simulink model "NavigationRocketPlant"  (R2025b)
settings: Solver=ode5  StartTime=0.0  StopTime=350  RelTol=1e-3
PostLoadFcn:
  | addpath('settings/')
  | addpath('settings/environment/')
  | 
  | run sensorSettings.m
InitFcn:
  | run(fullfile(fileparts(get_param(bdroot,'FileName')),'..','rocketPlantMain.m'))
values from neighbouring files (symbols this model uses):
  ba0 = zeros(3,1)    [rocketPlantMain.m]
  bg0 = zeros(3,1)    [rocketPlantMain.m]
  LLA0 = [Rocket.Latitude; Rocket.Longitude; Rocket.AltitudeMSL]    [rocketPlantMain.m]
  p0 = zeros(3,1)    [rocketPlantMain.m]
  P0 = zeros(15,15)    [rocketPlantMain.m]
  q0 = RocketInitialState(7:10)    [rocketPlantMain.m]
  RocketInitialState = rocketPlantInitialize(Rocket)    [rocketPlantMain.m]
  stationaryTime = Rocket.IgnitionTime    [rocketPlantMain.m]
  v0 = zeros(3,1)    [rocketPlantMain.m]
undefined symbols (not defined in the file or in its folder): DiscIntNeverNeededParam, dspblkCoreblockFVToolHelper, Environment, gcbh, GNSSConfig, GNSSInitialState, MEKF, pressure0, Rocket, Sensor, Weather
libraries: simulink x2, dspmathops x1
(part 1 of 3)
settings Model: Creator=wujia  LastModifiedBy=wujia

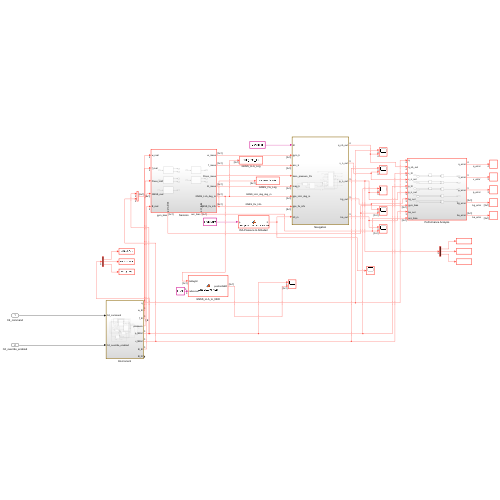
[thumbnail: Simulink's stored preview of the top-level diagram]
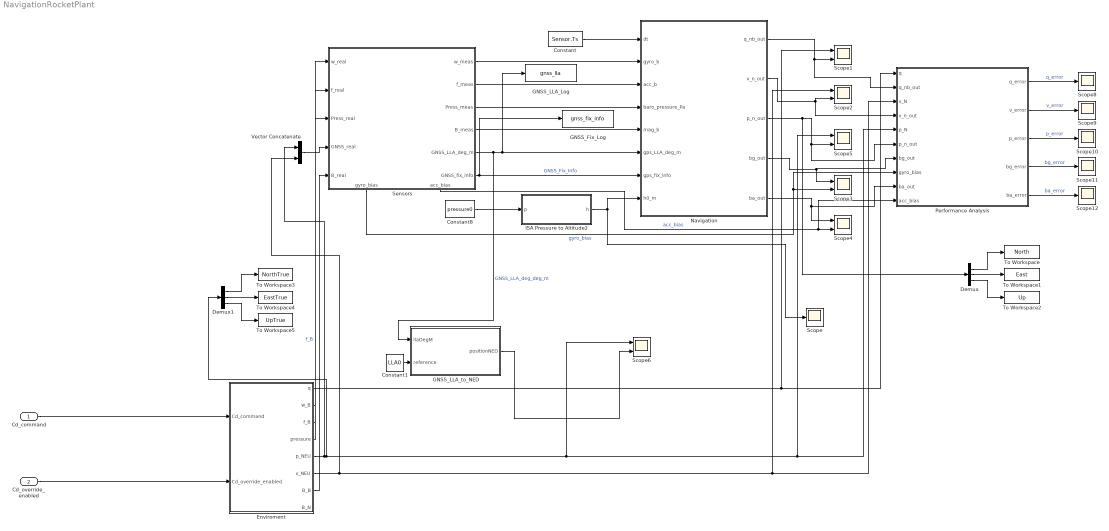
== system NavigationRocketPlant ==
  Cd_command : Inport  OutDataTypeStr=double  PortDimensions=1  SampleTime=Rocket.Ts  Interpolate=off
  Cd_override_enabled : Inport  Port=2  OutDataTypeStr=double  PortDimensions=1  SampleTime=Rocket.Ts  Interpolate=off
  Constant : Constant  Value=Sensor.Ts
  Constant1 : Constant  Value=LLA0
  Constant8 : Constant  Value=pressure0
  Demux : Demux  Outputs=3
  Demux1 : Demux  Outputs=3
  Enviroment : Subsystem
  GNSS_Fix_Log : ToWorkspace  VariableName=gnss_fix_info  SaveFormat=Timeseries  SampleTime=-1
  GNSS_LLA_Log : ToWorkspace  VariableName=gnss_lla  SaveFormat=Timeseries  SampleTime=-1
  GNSS_LLA_to_NED : MATLAB Function  TreatAsAtomicUnit=on
  ISA Pressure to Altitude2 : MATLAB Function  TreatAsAtomicUnit=on
  Navigation : Subsystem
  Performance Analysis : Subsystem
  Scope{,8..12} (6 alike) : Scope
      Scope settings: ActiveDisplayYMinimum=-1  ActiveDisplayYMaximum=1  DataLoggingVariableName=ScopeData18
      Scope10 settings: ActiveDisplayYMinimum=-43.238898122556691  ActiveDisplayYMaximum=55.159382964966909  DataLoggingVariableName=ScopeData12
      Scope11 settings: ActiveDisplayYMinimum=-0.047372671781054559  ActiveDisplayYMaximum=0.023017615287449465  DataLoggingVariableName=ScopeData13
      Scope12 settings: ActiveDisplayYMinimum=-0.56247304441899837  ActiveDisplayYMaximum=1.1440559822181913  DataLoggingVariableName=ScopeData14
      Scope8 settings: ActiveDisplayYMinimum=-2.4024992579145321  ActiveDisplayYMaximum=2.4014240203083954  DataLoggingVariableName=ScopeData6
      Scope9 settings: ActiveDisplayYMinimum=-73.4449521246089  ActiveDisplayYMaximum=67.234314688531754  DataLoggingVariableName=ScopeData8
  Scope{1..6} (6 alike) : Scope  NumInputPorts=2
      Scope1 settings: ActiveDisplayYMinimum=-1.2880369168448469  ActiveDisplayYMaximum=1.3322786485025644
      Scope2 settings: ActiveDisplayYMinimum=-66.391402806495847  ActiveDisplayYMaximum=368.05030772718362  DataLoggingVariableName=ScopeData2
      Scope3 settings: ActiveDisplayYMinimum=-0.019866552939701122  ActiveDisplayYMaximum=0.055696216205846576  DataLoggingVariableName=ScopeData3
      Scope4 settings: ActiveDisplayYMinimum=-0.56108731493308794  ActiveDisplayYMaximum=1.1446707904167028  DataLoggingVariableName=ScopeData4
      Scope5 settings: ActiveDisplayYMinimum=-703.59600028849377  ActiveDisplayYMaximum=4675.4737500320552  DataLoggingVariableName=ScopeData5
      Scope6 settings: ActiveDisplayYMinimum=-4.2977064407464418  ActiveDisplayYMaximum=41.562392937860714  DataLoggingVariableName=ScopeData7
  Sensors : Subsystem
      settings: PortSchema="{\"entries\":[{\"content\":{\"sides\":[{\"content\":{\"connectorIds\":[\"In1\",\"In2\",\"In3\",\"In4\",\"In5\"]},\"type\":\"ConnectorPlacement.EquallySpacedRectSide\",\"uuid\":\"7549c628-8b7d-407c-a68e-245c0e15f536\"},{\"content\":{\"connectorIds\":[\"Out1\",\"Out2\",\"Out3\",\"Out4\",\"Out5\",\"Out6\"],\"side\":\"RIGHT\"},\"type\":\"ConnectorPlacement.EquallySpacedRectSide\",\"uuid\":\"d27d0e7f-3d86-4e84-80b8-20c86293b7bf\"},{\"content\":{\"side\":\"TOP\"},\"type\":\"ConnectorPlacement.EquallySpacedRectSide\",\"uuid\":\"44c73c2c-96b0-4d3a-9d50-da6ca6099998\"},{\"content\":{\"connectorIds\":[\"Out7\",\"Out8\"],\"side\":\"BOTTOM\"},\"type\":\"ConnectorPlacement.EquallySpacedRectSide\",\"uuid\":\"8107c7d0-06da-4640-bff8-8544b9179788\"}]},\"type\":\"ConnectorPlacement.EquallySpacedConnector\",\"uuid\":\"f9c24899-cf40-457b-80ff-0dc7874e17ca\"}],\"packageUris\":[\"http://schema.mathworks.com/mf0/Connector/R2020b\"],\"version\":\"1.0\"}"
  To Workspace : ToWorkspace  VariableName=North  SaveFormat=Structure  SampleTime=-1
      settings: Save2DSignal=2-D array (concatenate along first dimension)
  To Workspace1 : ToWorkspace  VariableName=East  SaveFormat=Structure  SampleTime=-1
      settings: Save2DSignal=2-D array (concatenate along first dimension)
  To Workspace2 : ToWorkspace  VariableName=Up  SaveFormat=Structure  SampleTime=-1
      settings: Save2DSignal=2-D array (concatenate along first dimension)
  To Workspace3 : ToWorkspace  VariableName=NorthTrue  SaveFormat=Structure  SampleTime=-1
      settings: Save2DSignal=2-D array (concatenate along first dimension)
  To Workspace4 : ToWorkspace  VariableName=EastTrue  SaveFormat=Structure  SampleTime=-1
      settings: Save2DSignal=2-D array (concatenate along first dimension)
  To Workspace5 : ToWorkspace  VariableName=UpTrue  SaveFormat=Structure  SampleTime=-1
      settings: Save2DSignal=2-D array (concatenate along first dimension)
  Vector Concatenate : Concatenate  Mode=Multidimensional array
  wires:
  Sensors/4(B_meas) -> Navigation/5(mag_b)
  Sensors/3(Press_meas) -> Navigation/4(baro_pressure_Pa)
  Constant8/1 -> ISA Pressure to Altitude2/1(p)
  Sensors/7(gyro_bias) -> Performance Analysis/8(gyro_bias), Scope3/2  "gyro_bias"
  Sensors/8(acc_bias) -> Performance Analysis/10(acc_bias), Scope4/2  "acc_bias"
  Sensors/1(w_meas) -> Navigation/2(gyro_b)
  Constant/1 -> Navigation/1(dt)
  ISA Pressure to Altitude2/1(h) -> Scope/1, Navigation/8(h0_m)
  Navigation/1(q_nb_out) -> Performance Analysis/2(q_nb_out), Scope1/2
  Navigation/4(bg_out) -> Performance Analysis/7(bg_out), Scope3/1
  Navigation/5(ba_out) -> Scope4/1, Performance Analysis/9(ba_out)
  Vector Concatenate/1 -> Sensors/4(GNSS_real)
  Performance Analysis/1(q_error) -> Scope8/1  "q_error"
  Performance Analysis/2(v_error) -> Scope9/1  "v_error"
  Performance Analysis/5(ba_error) -> Scope12/1  "ba_error"
  Performance Analysis/4(bg_error) -> Scope11/1  "bg_error"
  Performance Analysis/3(p_error) -> Scope10/1  "p_error"
  Sensors/2(f_meas) -> Navigation/3(acc_b)
  Demux/1 -> To Workspace/1
  Demux/3 -> To Workspace2/1
  Demux/2 -> To Workspace1/1
  Demux1/1 -> To Workspace3/1
  Demux1/2 -> To Workspace4/1
  Demux1/3 -> To Workspace5/1
  Navigation/2(v_n_out) -> Performance Analysis/4(v_n_out), Scope2/2
  Navigation/3(p_n_out) -> Demux/1, Performance Analysis/6(p_n_out), Scope5/2
  Sensors/6(GNSS_fix_info) -> GNSS_Fix_Log/1, Navigation/7(gps_fix_info)  "GNSS_Fix_Info"
  Constant1/1 -> GNSS_LLA_to_NED/2(reference)
  GNSS_LLA_to_NED/1(positionNED) -> Scope6/2
  Sensors/5(GNSS_LLA_deg_m) -> Navigation/6(gps_LLA_deg_m), GNSS_LLA_Log/1, GNSS_LLA_to_NED/1(llaDegM)  "GNSS_LLA_deg_deg_m"
  Enviroment/2(w_B) -> Sensors/1(w_real)
  Enviroment/3(f_B) -> Sensors/2(f_real)  "f_B"
  Enviroment/7(B_B) -> Sensors/5(B_real)
  Enviroment/4(pressure) -> Sensors/3(Press_real)
  Enviroment/6(v_NEU) -> Performance Analysis/3(v_N), Scope2/1, Vector Concatenate/2
  Enviroment/1(q) -> Performance Analysis/1(q), Scope1/1
  Enviroment/5(p_NEU) -> Performance Analysis/5(p_N), Scope5/1, Scope6/1, Demux1/1, Vector Concatenate/1
  Cd_command/1 -> Enviroment/1(Cd_command)
  Cd_override_enabled/1 -> Enviroment/2(Cd_override_enabled)

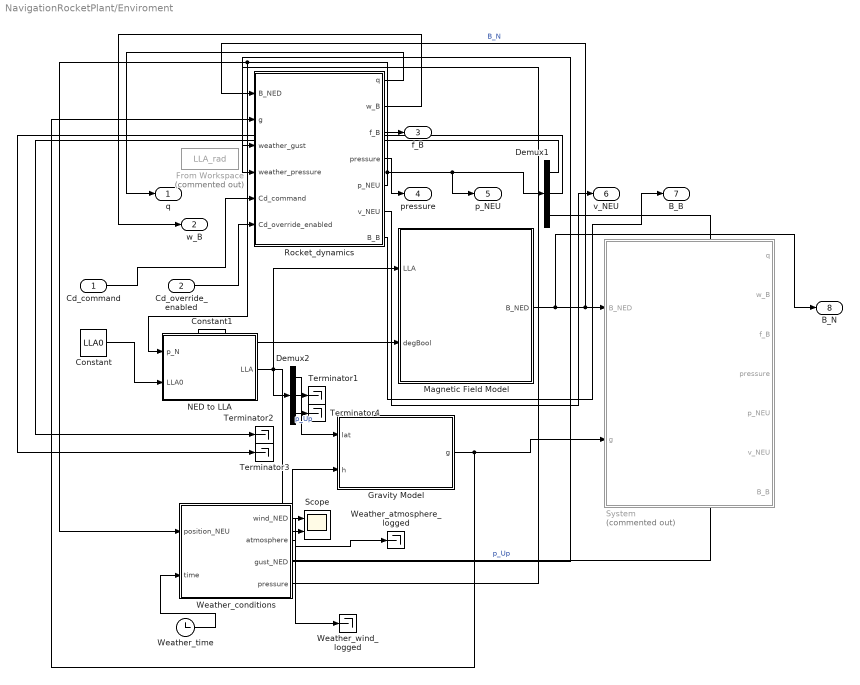
== system NavigationRocketPlant/Enviroment ==
  Cd_command : Inport  PortDimensions=1  SampleTime=Rocket.Ts
  Cd_override_enabled : Inport  Port=2  PortDimensions=1  SampleTime=Rocket.Ts
  Constant : Constant  Value=LLA0  VectorParams1D=off
  Constant1 : Constant  Value=0
  Demux1 : Demux  Outputs=3
  Demux2 : Demux  Outputs=3
  From Workspace : FromWorkspace  Commented=on  VariableName=LLA_rad
  Gravity Model : Subsystem
  Magnetic Field Model : Subsystem
  NED to LLA : MATLAB Function  TreatAsAtomicUnit=on
  Rocket_dynamics : Subsystem
  Scope : Scope  NumInputPorts=2
      settings: ActiveDisplayYMinimum=-1  ActiveDisplayYMaximum=1  DataLoggingVariableName=ScopeData9
  System : Subsystem  Description=Preserved CSV reference; inactive in physics-driven model. Original CSV model remains in the recovery artifact.  Commented=on
  Terminator{1..4} (4 alike) : Terminator
  Weather_atmosphere_logged : Terminator
  Weather_conditions : Subsystem
  Weather_time : Clock
  Weather_wind_logged : Terminator
  q : Outport
  w_B : Outport  Port=2
  f_B : Outport  Port=3
  pressure : Outport  Port=4
  p_NEU : Outport  Port=5
  v_NEU : Outport  Port=6
  B_B : Outport  Port=7
  B_N : Outport  Port=8
  wires:
  Demux2/2 -> Terminator1/1
  Demux2/3 -> Terminator4/1  "p_Up"
  Demux2/1 -> Gravity Model/1(lat)
  Demux1/3 -> Gravity Model/2(h)  "p_Up"
  Demux1/1 -> Terminator2/1
  Demux1/2 -> Terminator3/1
  Weather_conditions/2(atmosphere) -> Weather_atmosphere_logged/1
  Cd_override_enabled/1 -> Rocket_dynamics/6(Cd_override_enabled)
  Cd_command/1 -> Rocket_dynamics/5(Cd_command)
  Rocket_dynamics/7(B_B) -> B_B/1
  Rocket_dynamics/6(v_NEU) -> v_NEU/1
  Rocket_dynamics/5(p_NEU) -> Demux1/1, p_NEU/1, NED to LLA/1(p_N), Weather_conditions/1(position_NEU)
  Rocket_dynamics/4(pressure) -> pressure/1
  Rocket_dynamics/3(f_B) -> f_B/1
  Rocket_dynamics/2(w_B) -> w_B/1
  Rocket_dynamics/1(q) -> q/1
  Gravity Model/1(g) -> Rocket_dynamics/2(g), System/2(g)
  Magnetic Field Model/1(B_NED) -> Rocket_dynamics/1(B_NED), System/1(B_NED), B_N/1  "B_N"
  Weather_time/1 -> Weather_conditions/2(time)
  Weather_conditions/3(gust_NED) -> Rocket_dynamics/3(weather_gust)
  Weather_conditions/4(pressure) -> Rocket_dynamics/4(weather_pressure)
  Weather_conditions/1(wind_NED) -> Weather_wind_logged/1
  NED to LLA/1(LLA) -> Scope/2, Scope/1, Magnetic Field Model/1(LLA), Demux2/1
  Constant/1 -> NED to LLA/2(LLA0)
  Constant1/1 -> Magnetic Field Model/2(degBool)

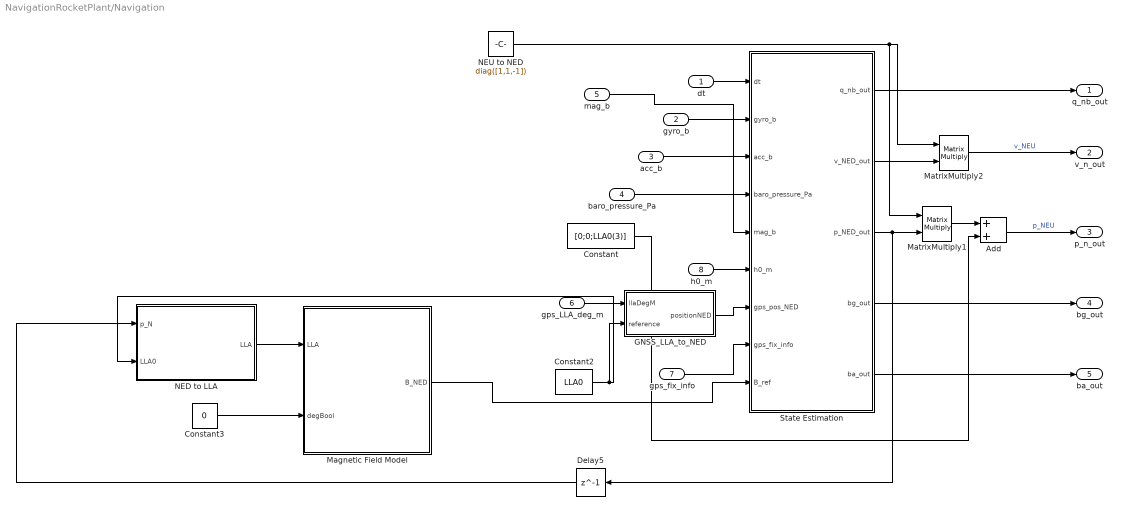
== system NavigationRocketPlant/Navigation ==
  dt : Inport
  gyro_b : Inport  Port=2
  acc_b : Inport  Port=3
  baro_pressure_Pa : Inport  Port=4
  mag_b : Inport  Port=5
  gps_LLA_deg_m : Inport  Port=6
  gps_fix_info : Inport  Port=7
  h0_m : Inport  Port=8
  Add : Sum
  Constant : Constant  Value=[0;0;LLA0(3)]
  Constant2 : Constant  Value=LLA0
  Constant3 : Constant  Value=0
  Delay5 : Delay  DelayLength=1  InitialCondition=p0
  GNSS_LLA_to_NED : MATLAB Function  TreatAsAtomicUnit=on
  Magnetic Field Model : Subsystem
  MatrixMultiply1 : Product  Multiplication=Matrix(*)
  MatrixMultiply2 : Product  Multiplication=Matrix(*)
  NED to LLA : MATLAB Function  TreatAsAtomicUnit=on
  NEU to NED : Constant  Value=diag([1,1,-1])
  State Estimation : Subsystem
  q_nb_out : Outport
  v_n_out : Outport  Port=2
  p_n_out : Outport  Port=3
  bg_out : Outport  Port=4
  ba_out : Outport  Port=5
  wires:
  MatrixMultiply2/1 -> v_n_out/1  "v_NEU"
  MatrixMultiply1/1 -> Add/1
  Constant3/1 -> Magnetic Field Model/2(degBool)
  NED to LLA/1(LLA) -> Magnetic Field Model/1(LLA)
  Delay5/1 -> NED to LLA/1(p_N)
  Add/1 -> p_n_out/1  "p_NEU"
  Constant/1 -> Add/2
  NEU to NED/1 -> MatrixMultiply2/1, MatrixMultiply1/1
  gps_fix_info/1 -> State Estimation/8(gps_fix_info)
  GNSS_LLA_to_NED/1(positionNED) -> State Estimation/7(gps_pos_NED)
  gps_LLA_deg_m/1 -> GNSS_LLA_to_NED/1(llaDegM)
  mag_b/1 -> State Estimation/5(mag_b)
  Constant2/1 -> GNSS_LLA_to_NED/2(reference), NED to LLA/2(LLA0)
  State Estimation/5(ba_out) -> ba_out/1
  State Estimation/4(bg_out) -> bg_out/1
  State Estimation/3(p_NED_out) -> MatrixMultiply1/2, Delay5/1
  State Estimation/2(v_NED_out) -> MatrixMultiply2/2
  State Estimation/1(q_nb_out) -> q_nb_out/1
  dt/1 -> State Estimation/1(dt)
  acc_b/1 -> State Estimation/3(acc_b)
  gyro_b/1 -> State Estimation/2(gyro_b)
  h0_m/1 -> State Estimation/6(h0_m)
  baro_pressure_Pa/1 -> State Estimation/4(baro_pressure_Pa)
  Magnetic Field Model/1(B_NED) -> State Estimation/9(B_ref)

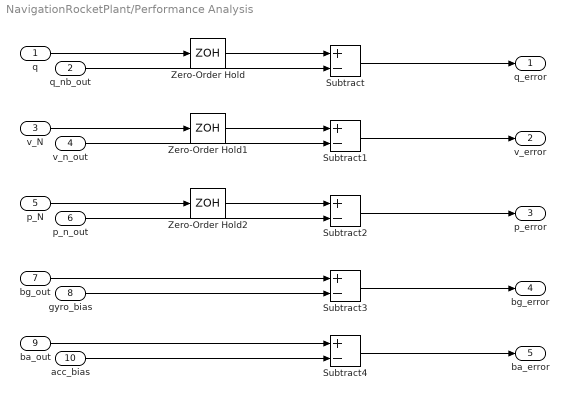
== system NavigationRocketPlant/Performance Analysis ==
  q : Inport
  q_nb_out : Inport  Port=2
  v_N : Inport  Port=3
  v_n_out : Inport  Port=4
  p_N : Inport  Port=5
  p_n_out : Inport  Port=6
  bg_out : Inport  Port=7
  gyro_bias : Inport  Port=8
  ba_out : Inport  Port=9
  acc_bias : Inport  Port=10
  Subtract{,1..4} (5 alike) : Sum  Inputs=+-
  Zero-Order Hold : ZeroOrderHold  SampleTime=Sensor.Ts
  Zero-Order Hold1 : ZeroOrderHold  SampleTime=-1
  Zero-Order Hold2 : ZeroOrderHold  SampleTime=-1
  q_error : Outport
  v_error : Outport  Port=2
  p_error : Outport  Port=3
  bg_error : Outport  Port=4
  ba_error : Outport  Port=5
  wires:
  q/1 -> Zero-Order Hold/1
  q_nb_out/1 -> Subtract/2
  v_n_out/1 -> Subtract1/2
  v_N/1 -> Zero-Order Hold1/1
  p_n_out/1 -> Subtract2/2
  p_N/1 -> Zero-Order Hold2/1
  bg_out/1 -> Subtract3/1
  gyro_bias/1 -> Subtract3/2
  ba_out/1 -> Subtract4/1
  acc_bias/1 -> Subtract4/2
  Zero-Order Hold1/1 -> Subtract1/1
  Zero-Order Hold2/1 -> Subtract2/1
  Subtract/1 -> q_error/1
  Subtract1/1 -> v_error/1
  Subtract2/1 -> p_error/1
  Subtract3/1 -> bg_error/1
  Subtract4/1 -> ba_error/1
  Zero-Order Hold/1 -> Subtract/1

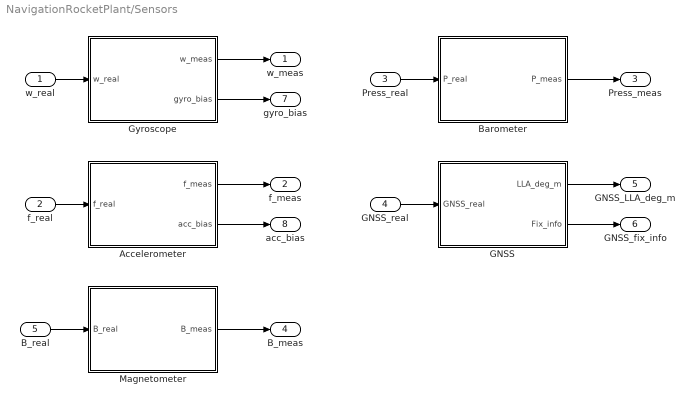
== system NavigationRocketPlant/Sensors ==
  w_real : Inport
  f_real : Inport  Port=2
  Press_real : Inport  Port=3
  GNSS_real : Inport  Port=4
  B_real : Inport  Port=5
  Accelerometer : Subsystem
  Barometer : Subsystem
  GNSS : Subsystem
  Gyroscope : Subsystem
  Magnetometer : Subsystem
  w_meas : Outport
  f_meas : Outport  Port=2
  Press_meas : Outport  Port=3
  B_meas : Outport  Port=4
  GNSS_LLA_deg_m : Outport  Description=Latitude [deg], longitude [deg], ellipsoid height [m].  Port=5
  GNSS_fix_info : Outport  Description=Fresh/valid/time/age/metric covariance/status; no velocity output.  Port=6
  gyro_bias : Outport  Port=7
  acc_bias : Outport  Port=8
  wires:
  B_real/1 -> Magnetometer/1(B_real)
  Magnetometer/1(B_meas) -> B_meas/1
  w_real/1 -> Gyroscope/1(w_real)
  f_real/1 -> Accelerometer/1(f_real)
  Accelerometer/1(f_meas) -> f_meas/1
  Gyroscope/1(w_meas) -> w_meas/1
  Barometer/1(P_meas) -> Press_meas/1
  Press_real/1 -> Barometer/1(P_real)
  GNSS_real/1 -> GNSS/1(GNSS_real)
  GNSS/1(LLA_deg_m) -> GNSS_LLA_deg_m/1
  GNSS/2(Fix_info) -> GNSS_fix_info/1
  Accelerometer/2(acc_bias) -> acc_bias/1
  Gyroscope/2(gyro_bias) -> gyro_bias/1

== system NavigationRocketPlant/Enviroment/Gravity Model ==
  lat : Inport
  h : Inport  Port=2
  MATLAB Function : MATLAB Function  TreatAsAtomicUnit=on
  MATLAB Function1 : MATLAB Function  TreatAsAtomicUnit=on
  Scope : Scope  NumInputPorts=2
      settings: ActiveDisplayYMinimum=9.7899742881861069  ActiveDisplayYMaximum=9.8055275433313476  DataLoggingVariableName=ScopeData19
  g : Outport
  wires:
  MATLAB Function/1(g) -> Scope/1
  h/1 -> MATLAB Function1/1(h), MATLAB Function/1(h)
  lat/1 -> MATLAB Function1/2(lat)
  MATLAB Function1/1(g_n) -> Scope/2, g/1

== system NavigationRocketPlant/Enviroment/Magnetic Field Model ==
  LLA : Inport
  degBool : Inport  Port=2
  Constant : Constant  Value=13
  MATLAB Function1 : MATLAB Function  Commented=on  TreatAsAtomicUnit=on
  Magnetic Field Model : MATLAB Function  TreatAsAtomicUnit=on
  Terminator : Terminator
  Terminator1 : Terminator
  g : Constant  Value=Environment.IGRF13.g
  h : Constant  Value=Environment.IGRF13.h
  order : Constant  Value=Environment.IGRF13.order
  B_NED : Outport
  wires:
  Magnetic Field Model/1(B_ECEF) -> Terminator1/1
  Magnetic Field Model/2(B_NED) -> B_NED/1
  g/1 -> Magnetic Field Model/2(g)
  order/1 -> ?
  h/1 -> Magnetic Field Model/3(h)
  LLA/1 -> Magnetic Field Model/1(LLA)
  Magnetic Field Model/3(B_sph) -> Terminator/1
  degBool/1 -> Magnetic Field Model/7(degBool)
  Constant/1 -> Magnetic Field Model/4(Nmax)

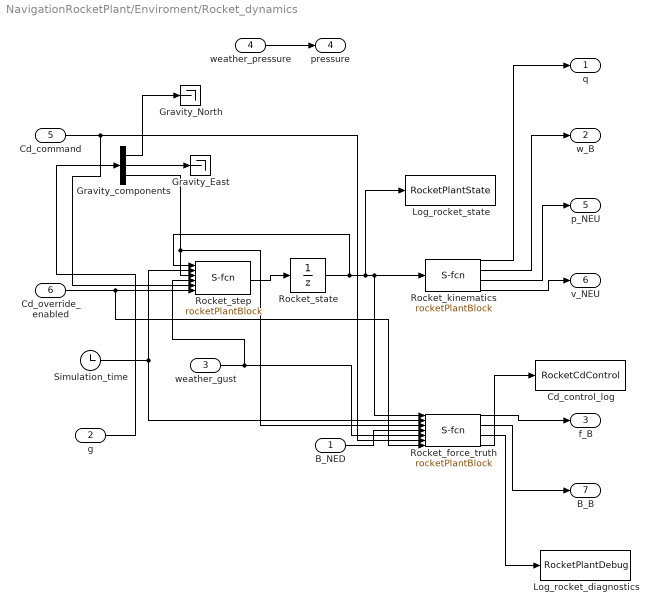
== system NavigationRocketPlant/Enviroment/Rocket_dynamics ==
  B_NED : Inport
  g : Inport  Port=2
  weather_gust : Inport  Port=3
  weather_pressure : Inport  Port=4
  Cd_command : Inport  Port=5  PortDimensions=1  SampleTime=Rocket.Ts
  Cd_override_enabled : Inport  Port=6  PortDimensions=1  SampleTime=Rocket.Ts
  Cd_control_log : ToWorkspace  VariableName=RocketCdControl  SaveFormat=Timeseries  SampleTime=-1
  Gravity_East : Terminator
  Gravity_North : Terminator
  Gravity_components : Demux  Outputs=3
  Log_rocket_diagnostics : ToWorkspace  VariableName=RocketPlantDebug  SaveFormat=Timeseries  SampleTime=-1
  Log_rocket_state : ToWorkspace  VariableName=RocketPlantState  SaveFormat=Timeseries  SampleTime=-1
  Rocket_force_truth : M-S-Function  FunctionName=rocketPlantBlock  Parameters=Rocket,3,Weather
  Rocket_kinematics : M-S-Function  FunctionName=rocketPlantBlock  Parameters=Rocket,2,Weather
  Rocket_state : UnitDelay  InitialCondition=RocketInitialState  SampleTime=Rocket.Ts  HasFrameUpgradeWarning=on
  Rocket_step : M-S-Function  FunctionName=rocketPlantBlock  Parameters=Rocket,1,Weather
  Simulation_time : Clock
  q : Outport
  w_B : Outport  Port=2
  f_B : Outport  Port=3
  pressure : Outport  Port=4
  p_NEU : Outport  Port=5
  v_NEU : Outport  Port=6
  B_B : Outport  Port=7
  wires:
  Rocket_force_truth/3 -> Log_rocket_diagnostics/1
  Rocket_force_truth/2 -> B_B/1
  Rocket_force_truth/1 -> f_B/1
  Rocket_kinematics/4 -> v_NEU/1
  Rocket_kinematics/3 -> p_NEU/1
  Rocket_kinematics/2 -> w_B/1
  Rocket_kinematics/1 -> q/1
  B_NED/1 -> Rocket_force_truth/4
  Rocket_step/1 -> Rocket_state/1
  g/1 -> Gravity_components/1
  Simulation_time/1 -> Rocket_step/2, Rocket_force_truth/2
  Rocket_state/1 -> Rocket_kinematics/1, Rocket_force_truth/1, Log_rocket_state/1, Rocket_step/1
  Gravity_components/3 -> Rocket_force_truth/3, Rocket_step/3
  Gravity_components/2 -> Gravity_East/1
  Gravity_components/1 -> Gravity_North/1
  weather_pressure/1 -> pressure/1
  weather_gust/1 -> Rocket_step/4, Rocket_force_truth/5
  Rocket_force_truth/4 -> Cd_control_log/1
  Cd_override_enabled/1 -> Rocket_force_truth/7, Rocket_step/6
  Cd_command/1 -> Rocket_force_truth/6, Rocket_step/5

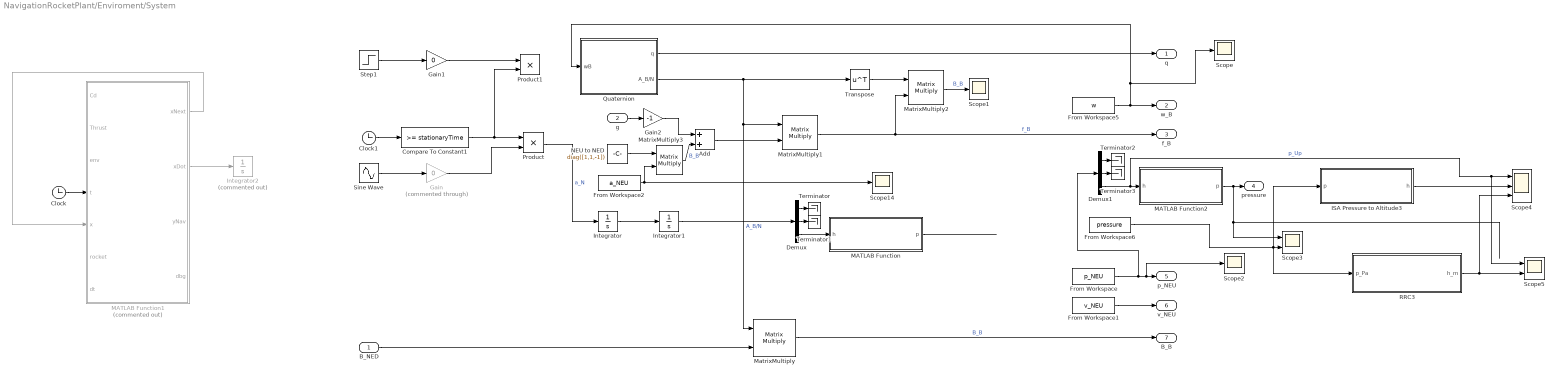
== system NavigationRocketPlant/Enviroment/System ==
  B_NED : Inport
  g : Inport  Port=2
  Add : Sum
  Clock : Clock
  Clock1 : Clock
  Compare To Constant1 : simulink/Logic and Bit Operations/Compare To Constant  relop=>=  const=stationaryTime  OutDataTypeStr=uint8
  Demux : Demux  Outputs=3
  Demux1 : Demux  Outputs=3
  From Workspace : FromWorkspace  VariableName=p_NEU  SampleTime=0.02
  From Workspace1 : FromWorkspace  VariableName=v_NEU  SampleTime=0.02
  From Workspace2 : FromWorkspace  VariableName=a_NEU  SampleTime=0.02
  From Workspace5 : FromWorkspace  VariableName=w  SampleTime=0.02
  From Workspace6 : FromWorkspace  VariableName=pressure  SampleTime=0.02
  Gain : Gain  Commented=through  Gain=0
  Gain1 : Gain  Gain=0
  Gain2 : Gain  Gain=-1
  ISA Pressure to Altitude3 : MATLAB Function  TreatAsAtomicUnit=on
  Integrator : Integrator  InitialCondition=v0
  Integrator1 : Integrator  InitialCondition=p0
  Integrator2 : Integrator  Commented=on
  MATLAB Function : MATLAB Function  TreatAsAtomicUnit=on
  MATLAB Function1 : MATLAB Function  Commented=on  TreatAsAtomicUnit=on
  MATLAB Function2 : MATLAB Function  TreatAsAtomicUnit=on
  MatrixMultiply{,1..3} (4 alike) : Product  Multiplication=Matrix(*)
  NEU to NED : Constant  Value=diag([1,1,-1])
  Product : Product
  Product1 : Product
  "Quaternion " : Subsystem
  RRC3 : MATLAB Function  TreatAsAtomicUnit=on
  Scope{,1..2,14} (4 alike) : Scope
      Scope settings: ActiveDisplayYMinimum=-1.6045475791322781E-7  ActiveDisplayYMaximum=2.6814536853544749E-7
      Scope1 settings: ActiveDisplayYMinimum=-185.19167567929276  ActiveDisplayYMaximum=161.84122591706938  DataLoggingVariableName=ScopeData15
      Scope14 settings: ActiveDisplayYMinimum=-34.139290674344366  ActiveDisplayYMaximum=25.55163695065562  DataLoggingVariableName=ScopeData20
      Scope2 settings: ActiveDisplayYMinimum=-1  ActiveDisplayYMaximum=1  DataLoggingVariableName=ScopeData16
  Scope3 : Scope  NumInputPorts=2
      settings: ActiveDisplayYMinimum=56252.912155082136  ActiveDisplayYMaximum=99152.104181642775  DataLoggingVariableName=ScopeData17
  Scope4 : Scope  NumInputPorts=3
      settings: ActiveDisplayYMinimum=3919.4855259572764  ActiveDisplayYMaximum=3932.9364289417367  DataLoggingVariableName=ScopeData17
  Scope5 : Scope  NumInputPorts=2
      settings: ActiveDisplayYMinimum=496.42915312500008  ActiveDisplayYMaximum=4542.137621875  DataLoggingVariableName=ScopeData11
  Sine Wave : Sin  Amplitude=[1;1;1]  Frequency=[0.1;0.2;0.3]  SampleTime=0  VectorParams1D=off
  Step1 : Step  Time=stationaryTime  After=[0.1;0.5;0.3]  SampleTime=0  VectorParams1D=off
  Terminator{,1..3} (4 alike) : Terminator
  Transpose : Math  Operator=transpose
  q : Outport
  w_B : Outport  Port=2
  f_B : Outport  Port=3
  pressure : Outport  Port=4
  p_NEU : Outport  Port=5
  v_NEU : Outport  Port=6
  B_B : Outport  Port=7
  wires:
  Integrator1/1 -> Demux/1
  B_NED/1 -> MatrixMultiply/2
  Clock1/1 -> Compare To Constant1/1
  Product/1 -> Integrator/1  "a_N"
  g/1 -> Gain2/1
  Step1/1 -> Gain1/1
  MatrixMultiply/1 -> B_B/1  "B_B"
  Integrator/1 -> Integrator1/1
  "Quaternion "/2("A_B/N ") -> Transpose/1, MatrixMultiply/1, MatrixMultiply1/1  "A_B/N"
  Compare To Constant1/1 -> Product1/2, Product/1
  Add/1 -> MatrixMultiply1/2
  Demux/1 -> Terminator/1
  Sine Wave/1 -> Gain/1
  Demux/3 -> MATLAB Function/1(h)
  MatrixMultiply1/1 -> MatrixMultiply2/2, f_B/1  "f_B"
  Gain/1 -> Product/2
  Demux/2 -> Terminator1/1
  MATLAB Function1/2(xDot) -> Integrator2/1
  From Workspace6/1 -> RRC3/1(p_Pa), ISA Pressure to Altitude3/1(p), Scope3/2
  From Workspace1/1 -> v_NEU/1
  From Workspace2/1 -> Scope14/1, MatrixMultiply3/2
  "Quaternion "/1(q) -> q/1
  Transpose/1 -> MatrixMultiply2/1
  MatrixMultiply2/1 -> Scope1/1  "B_B"
  Demux1/2 -> Terminator3/1
  Demux1/1 -> Terminator2/1
  MATLAB Function2/1(p) -> Scope3/1, pressure/1
  Gain1/1 -> Product1/1
  From Workspace/1 -> Demux1/1, p_NEU/1, Scope2/1
  From Workspace5/1 -> Scope/1, "Quaternion "/1(wB), w_B/1
  NEU to NED/1 -> MatrixMultiply3/1
  MatrixMultiply3/1 -> Add/2  "B_B"
  ISA Pressure to Altitude3/1(h) -> Scope4/2
  Demux1/3 -> Scope5/1, Scope4/1, MATLAB Function2/1(h)  "p_Up"
  RRC3/1(h_m) -> Scope4/3, Scope5/2
  Gain2/1 -> Add/1
  MATLAB Function1/1(xNext) -> MATLAB Function1/5(x)
  Clock/1 -> MATLAB Function1/4(t)
  MATLAB Function/1(p) -> ?

== system NavigationRocketPlant/Enviroment/Weather_conditions ==
  position_NEU : Inport
  time : Inport  Port=2
  Atmosphere_components : Demux  Outputs=5
  Density_log_only : Terminator
  Humidity_log_only : Terminator
  Log_weather_truth : ToWorkspace  VariableName=WeatherTruth  SaveFormat=Timeseries  SampleTime=-1
  Sound_speed_log_only : Terminator
  Temperature_log_only : Terminator
  Weather_log_vector : Mux  Inputs=3
  Weather_truth : M-S-Function  FunctionName=rocketWeatherBlock  Parameters=Rocket,Weather,Rocket.Ts
  wind_NED : Outport
  atmosphere : Outport  Port=2
  gust_NED : Outport  Port=3
  pressure : Outport  Port=4
  wires:
  Weather_truth/3 -> gust_NED/1, Weather_log_vector/3
  Weather_truth/2 -> Atmosphere_components/1, Weather_log_vector/2, atmosphere/1
  Weather_truth/1 -> Weather_log_vector/1, wind_NED/1
  time/1 -> Weather_truth/2
  position_NEU/1 -> Weather_truth/1
  Weather_log_vector/1 -> Log_weather_truth/1
  Atmosphere_components/1 -> Density_log_only/1
  Atmosphere_components/2 -> pressure/1
  Atmosphere_components/3 -> Sound_speed_log_only/1
  Atmosphere_components/4 -> Temperature_log_only/1
  Atmosphere_components/5 -> Humidity_log_only/1

== system NavigationRocketPlant/Navigation/Magnetic Field Model ==
  LLA : Inport
  degBool : Inport  Port=2
  Magnetic Field Model : MATLAB Function  TreatAsAtomicUnit=on
  Terminator : Terminator
  Terminator1 : Terminator
  g : Constant  Value=Environment.IGRF13.g
  h : Constant  Value=Environment.IGRF13.h
  order : Constant  Value=Environment.IGRF13.order
  B_NED : Outport
  wires:
  Magnetic Field Model/1(B_ECEF) -> Terminator1/1
  Magnetic Field Model/2(B_NED) -> B_NED/1
  g/1 -> Magnetic Field Model/2(g)
  order/1 -> Magnetic Field Model/4(Nmax)
  h/1 -> Magnetic Field Model/3(h)
  LLA/1 -> Magnetic Field Model/1(LLA)
  Magnetic Field Model/3(B_sph) -> Terminator/1
  degBool/1 -> Magnetic Field Model/5(degBool)

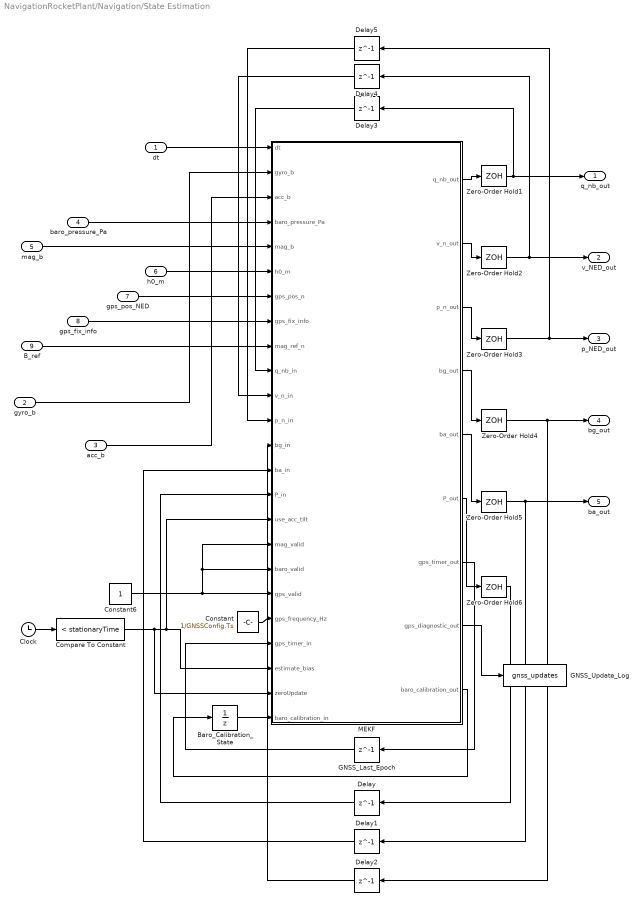
== system NavigationRocketPlant/Navigation/State Estimation ==
  dt : Inport
  gyro_b : Inport  Port=2
  acc_b : Inport  Port=3
  baro_pressure_Pa : Inport  Port=4
  mag_b : Inport  Port=5
  h0_m : Inport  Port=6
  gps_pos_NED : Inport  Port=7
  gps_fix_info : Inport  Port=8
  B_ref : Inport  Port=9
  Baro_Calibration_State : UnitDelay  InitialCondition=[0;0]  SampleTime=Sensor.Ts  HasFrameUpgradeWarning=on
  Clock : Clock
  Compare To Constant : simulink/Logic and Bit Operations/Compare To Constant  relop=<  const=stationaryTime  OutDataTypeStr=boolean
  Constant : Constant  Value=1/GNSSConfig.Ts
  Constant6 : Constant
  Delay : Delay  DelayLength=1  InitialCondition=P0  SampleTime=Sensor.Ts
  Delay1 : Delay  DelayLength=1  InitialCondition=ba0  SampleTime=Sensor.Ts
  Delay2 : Delay  DelayLength=1  InitialCondition=bg0  SampleTime=Sensor.Ts
  Delay3 : Delay  DelayLength=1  InitialCondition=q0  SampleTime=Sensor.Ts
  Delay4 : Delay  DelayLength=1  InitialCondition=v0  SampleTime=Sensor.Ts
  Delay5 : Delay  DelayLength=1  InitialCondition=p0  SampleTime=Sensor.Ts
  GNSS_Last_Epoch : Delay  DelayLength=1  InitialCondition=-1  InputProcessing=Columns as channels (frame based)
  GNSS_Update_Log : ToWorkspace  VariableName=gnss_updates  SaveFormat=Timeseries  SampleTime=-1
  MEKF : MATLAB Function  TreatAsAtomicUnit=on
  Zero-Order Hold{1..6} (6 alike) : ZeroOrderHold  SampleTime=-1
  q_nb_out : Outport
  v_NED_out : Outport  Port=2
  p_NED_out : Outport  Port=3
  bg_out : Outport  Port=4
  ba_out : Outport  Port=5
  wires:
  Clock/1 -> Compare To Constant/1
  Zero-Order Hold1/1 -> Delay3/1, q_nb_out/1
  Zero-Order Hold2/1 -> v_NED_out/1, Delay4/1
  Zero-Order Hold3/1 -> p_NED_out/1, Delay5/1
  Zero-Order Hold4/1 -> Delay2/1, bg_out/1
  Zero-Order Hold5/1 -> Delay1/1, ba_out/1
  Zero-Order Hold6/1 -> Delay/1
  Baro_Calibration_State/1 -> MEKF/24(baro_calibration_in)
  MEKF/9(baro_calibration_out) -> Baro_Calibration_State/1
  MEKF/8(gps_diagnostic_out) -> GNSS_Update_Log/1
  gyro_b/1 -> MEKF/2(gyro_b)
  acc_b/1 -> MEKF/3(acc_b)
  MEKF/6(P_out) -> Zero-Order Hold6/1
  Constant/1 -> MEKF/20(gps_frequency_Hz)
  GNSS_Last_Epoch/1 -> MEKF/21(gps_timer_in)
  MEKF/7(gps_timer_out) -> GNSS_Last_Epoch/1
  Delay1/1 -> MEKF/14(ba_in)
  Constant6/1 -> MEKF/17(mag_valid), MEKF/18(baro_valid), MEKF/19(gps_valid)
  Delay/1 -> MEKF/15(P_in)
  mag_b/1 -> MEKF/5(mag_b)
  Delay5/1 -> MEKF/12(p_n_in)
  MEKF/3(p_n_out) -> Zero-Order Hold3/1
  gps_pos_NED/1 -> MEKF/7(gps_pos_n)
  h0_m/1 -> MEKF/6(h0_m)
  baro_pressure_Pa/1 -> MEKF/4(baro_pressure_Pa)
  gps_fix_info/1 -> MEKF/8(gps_fix_info)
  B_ref/1 -> MEKF/9(mag_ref_n)
  MEKF/1(q_nb_out) -> Zero-Order Hold1/1
  dt/1 -> MEKF/1(dt)
  Compare To Constant/1 -> MEKF/16(use_acc_tilt), MEKF/22(estimate_bias), MEKF/23(zeroUpdate)
  Delay2/1 -> MEKF/13(bg_in)
  MEKF/4(bg_out) -> Zero-Order Hold4/1
  Delay4/1 -> MEKF/11(v_n_in)
  MEKF/5(ba_out) -> Zero-Order Hold5/1
  MEKF/2(v_n_out) -> Zero-Order Hold2/1
  Delay3/1 -> MEKF/10(q_nb_in)

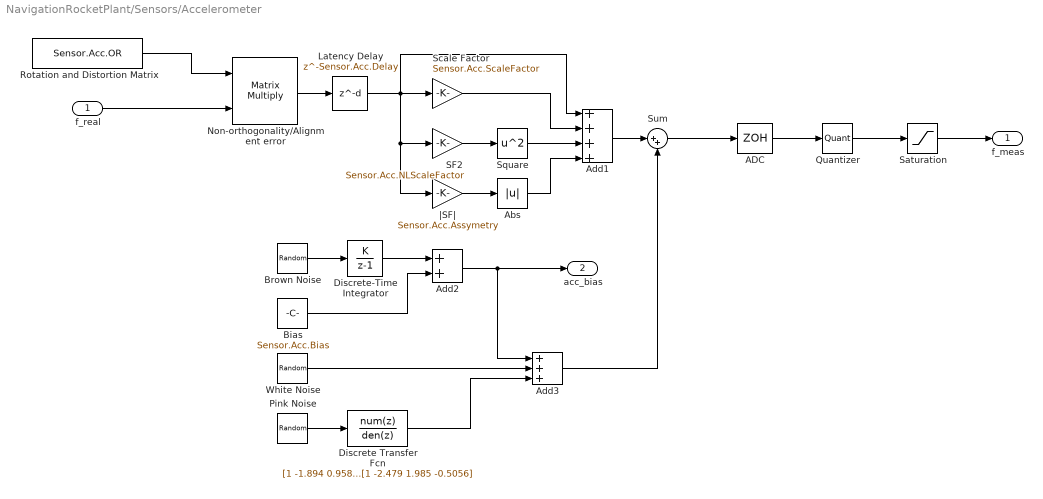
== system NavigationRocketPlant/Sensors/Accelerometer ==
  f_real : Inport
  ADC : ZeroOrderHold  SampleTime=Sensor.Acc.Ts
  Abs : Abs  SaturateOnIntegerOverflow=off
  Add1 : Sum  Inputs=++++
  Add2 : Sum
  Add3 : Sum  Inputs=+++
  Bias : Constant  Value=Sensor.Acc.Bias  VectorParams1D=off  SampleTime=Sensor.Acc.Ts
  Brown Noise : RandomNumber  Mean=Sensor.Acc.Noise.Brown.Mean  Variance=Sensor.Acc.Noise.Brown.Variance  Seed=Sensor.Acc.Noise.Brown.Seed  SampleTime=Sensor.Acc.Ts  VectorParams1D=off
  Discrete Transfer Fcn : DiscreteTransferFcn  LoadFcn=dspblkCoreblockFVToolHelper(gcbh,'load');  Numerator=[1 -1.894 0.9586 -0.06213]  Denominator=[1 -2.479 1.985 -0.5056]
      settings: CopyFcn=dspblkCoreblockFVToolHelper(gcbh,'copy');  DeleteFcn=dspblkCoreblockFVToolHelper(gcbh,'close');  ModelCloseFcn=dspblkCoreblockFVToolHelper(gcbh,'close');  PreSaveFcn=dspblkCoreblockFVToolHelper(gcbh,'presave');  PostSaveFcn=dspblkCoreblockFVToolHelper(gcbh,'postsave');  CloseFcn=dspblkCoreblockFVToolHelper(gcbh,'close');
  Discrete-Time Integrator : DiscreteIntegrator  IntegratorMethod=Accumulation: Forward Euler  SampleTime=Sensor.Acc.Ts  ICPrevOutput=DiscIntNeverNeededParam  ICPrevScaledInput=DiscIntNeverNeededParam
  Latency Delay : Delay  DelayLength=Sensor.Acc.Delay  SampleTime=Sensor.Acc.Ts
  Non-orthogonality/Alignment error : Product  Multiplication=Matrix(*)
  Pink Noise : RandomNumber  Mean=Sensor.Acc.Noise.Pink.Mean  Variance=Sensor.Acc.Noise.Pink.Variance  Seed=Sensor.Acc.Noise.Pink.Seed  SampleTime=Sensor.Acc.Ts  VectorParams1D=off
  Quantizer : Quantizer  QuantizationInterval=Sensor.Acc.Quant
  Rotation and Distortion Matrix : Constant  Value=Sensor.Acc.OR
  SF2 : Gain  Gain=Sensor.Acc.NLScaleFactor
  "Saturation " : Saturate  UpperLimit=Sensor.Acc.UpperLim  LowerLimit=Sensor.Acc.LowerLim
  Scale Factor : Gain  Gain=Sensor.Acc.ScaleFactor
  Square : Math  Operator=square
  Sum : Sum  Inputs=|++
  White Noise : RandomNumber  Mean=Sensor.Acc.Noise.White.Mean  Variance=Sensor.Acc.Noise.White.Variance  Seed=Sensor.Acc.Noise.White.Seed  SampleTime=Sensor.Acc.Ts  VectorParams1D=off
  |SF| : Gain  Gain=Sensor.Acc.Assymetry
  f_meas : Outport
  acc_bias : Outport  Port=2
  wires:
  f_real/1 -> Non-orthogonality/Alignment error/2
  Sum/1 -> ADC/1
  White Noise/1 -> Add3/2
  Bias/1 -> Add2/2
  Add3/1 -> Sum/2
  Brown Noise/1 -> Discrete-Time Integrator/1
  Discrete-Time Integrator/1 -> Add2/1
  ADC/1 -> Quantizer/1
  Latency Delay/1 -> Add1/1, SF2/1, |SF|/1, Scale Factor/1
  "Saturation "/1 -> f_meas/1
  Pink Noise/1 -> Discrete Transfer Fcn/1
  Discrete Transfer Fcn/1 -> Add3/3
  SF2/1 -> Square/1
  |SF|/1 -> Abs/1
  Scale Factor/1 -> Add1/2
  Square/1 -> Add1/3
  Abs/1 -> Add1/4
  Add1/1 -> Sum/1
  Quantizer/1 -> "Saturation "/1
  Non-orthogonality/Alignment error/1 -> Latency Delay/1
  Rotation and Distortion Matrix/1 -> Non-orthogonality/Alignment error/1
  Add2/1 -> acc_bias/1, Add3/1

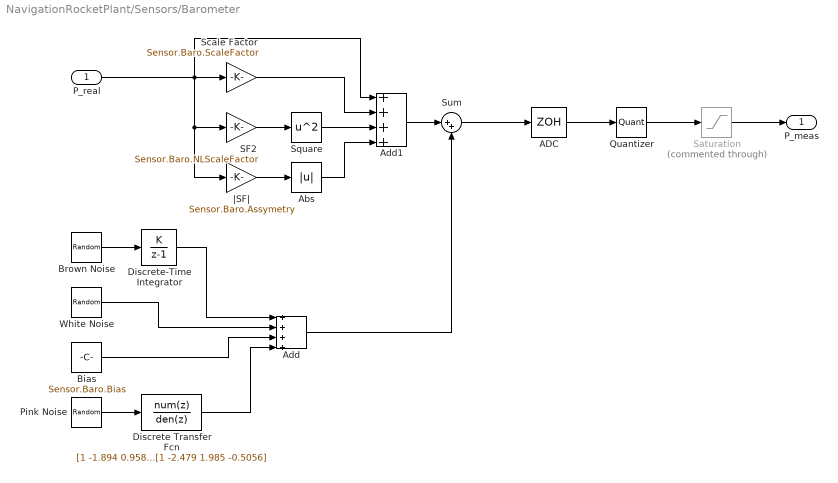
== system NavigationRocketPlant/Sensors/Barometer ==
  P_real : Inport
  ADC : ZeroOrderHold  SampleTime=Sensor.Baro.Ts
  Abs : Abs  SaturateOnIntegerOverflow=off
  Add : Sum  Inputs=++++
  Add1 : Sum  Inputs=++++
  Bias : Constant  Value=Sensor.Baro.Bias
  Brown Noise : RandomNumber  Mean=Sensor.Baro.Noise.Brown.Mean  Variance=Sensor.Baro.Noise.Brown.Variance  Seed=Sensor.Baro.Noise.Brown.Seed  SampleTime=Sensor.Baro.Ts
  Discrete Transfer Fcn : DiscreteTransferFcn  LoadFcn=dspblkCoreblockFVToolHelper(gcbh,'load');  Numerator=[1 -1.894 0.9586 -0.06213]  Denominator=[1 -2.479 1.985 -0.5056]
      settings: CopyFcn=dspblkCoreblockFVToolHelper(gcbh,'copy');  DeleteFcn=dspblkCoreblockFVToolHelper(gcbh,'close');  ModelCloseFcn=dspblkCoreblockFVToolHelper(gcbh,'close');  PreSaveFcn=dspblkCoreblockFVToolHelper(gcbh,'presave');  PostSaveFcn=dspblkCoreblockFVToolHelper(gcbh,'postsave');  CloseFcn=dspblkCoreblockFVToolHelper(gcbh,'close');
  Discrete-Time Integrator : DiscreteIntegrator  IntegratorMethod=Accumulation: Forward Euler  SampleTime=Sensor.Baro.Ts  ICPrevOutput=DiscIntNeverNeededParam  ICPrevScaledInput=DiscIntNeverNeededParam
  Pink Noise : RandomNumber  Mean=Sensor.Baro.Noise.Pink.Mean  Variance=Sensor.Baro.Noise.Pink.Variance  Seed=Sensor.Baro.Noise.Pink.Seed  SampleTime=Sensor.Baro.Ts
  Quantizer : Quantizer  QuantizationInterval=Sensor.Baro.Quant
  SF2 : Gain  Gain=Sensor.Baro.NLScaleFactor
  "Saturation " : Saturate  Commented=through  UpperLimit=Sensor.Baro.UpperLim  LowerLimit=Sensor.Baro.LowerLim
  Scale Factor : Gain  Gain=Sensor.Baro.ScaleFactor
  Square : Math  Operator=square
  Sum : Sum  Inputs=|++
  White Noise : RandomNumber  Mean=Sensor.Baro.Noise.White.Mean  Variance=Sensor.Baro.Noise.White.Variance  Seed=Sensor.Baro.Noise.White.Seed  SampleTime=Sensor.Baro.Ts
  |SF| : Gain  Gain=Sensor.Baro.Assymetry
  P_meas : Outport
  wires:
  Sum/1 -> ADC/1
  White Noise/1 -> Add/2
  Bias/1 -> Add/3
  Add/1 -> Sum/2
  Brown Noise/1 -> Discrete-Time Integrator/1
  Discrete-Time Integrator/1 -> Add/1
  ADC/1 -> Quantizer/1
  P_real/1 -> Add1/1, SF2/1, |SF|/1, Scale Factor/1
  "Saturation "/1 -> P_meas/1
  Pink Noise/1 -> Discrete Transfer Fcn/1
  Discrete Transfer Fcn/1 -> Add/4
  SF2/1 -> Square/1
  |SF|/1 -> Abs/1
  Scale Factor/1 -> Add1/2
  Square/1 -> Add1/3
  Abs/1 -> Add1/4
  Add1/1 -> Sum/1
  Quantizer/1 -> "Saturation "/1

== system NavigationRocketPlant/Sensors/GNSS ==
  GNSS_real : Inport
  GNSS_Clock : DigitalClock  SampleTime=GNSSConfig.Ts/GNSSConfig.TransportSubsteps
  GNSS_Consume : MATLAB Function  TreatAsAtomicUnit=on
  GNSS_Last_Delivery : UnitDelay  InitialCondition=-1  SampleTime=Sensor.Ts  HasFrameUpgradeWarning=on
  GNSS_Poll_Clock : DigitalClock  SampleTime=Sensor.Ts
  GNSS_Receiver : MATLAB Function  TreatAsAtomicUnit=on
  GNSS_Reference : Constant  Value=LLA0
  GNSS_Skipped_Log : ToWorkspace  VariableName=gnss_skipped_epochs  SaveFormat=Timeseries  SampleTime=-1
  GNSS_State : UnitDelay  InitialCondition=GNSSInitialState  SampleTime=GNSSConfig.Ts/GNSSConfig.TransportSubsteps  HasFrameUpgradeWarning=on
  GNSS_Truth_Sampling : ZeroOrderHold  SampleTime=GNSSConfig.Ts/GNSSConfig.TransportSubsteps
  GNSS_to_IMU : RateTransition  Deterministic=off  InitialCondition=[GNSSInitialState.heldLLA(1:2); GNSSInitialState.heldLLA(3)+GNSSConfig.GeoidSeparation; GNSSInitialState.heldInfo]  OutPortSampleTime=Sensor.Ts
  Receiver_Packet : Mux  Inputs=2
  LLA_deg_m : Outport  Description=Latitude [deg], longitude [deg], ellipsoid height [m].
  Fix_info : Outport  Description=[fresh; valid; acquisitionTime; age; sigmaN; sigmaE; sigmaD; reasonCode]  Port=2
  wires:
  GNSS_Truth_Sampling/1 -> GNSS_Receiver/1(truth_NEU)
  GNSS_real/1 -> GNSS_Truth_Sampling/1
  GNSS_Reference/1 -> GNSS_Receiver/3(reference)
  GNSS_Clock/1 -> GNSS_Receiver/2(time_s)
  GNSS_State/1 -> GNSS_Receiver/4(state_in)
  GNSS_Receiver/3(state_out) -> GNSS_State/1
  GNSS_Receiver/1(LLA_deg_m) -> Receiver_Packet/1
  GNSS_Receiver/2(fix_info) -> Receiver_Packet/2
  GNSS_Consume/2(fix_info) -> Fix_info/1
  GNSS_Consume/1(LLA_deg_m) -> LLA_deg_m/1
  GNSS_Consume/4(skipped_epochs) -> GNSS_Skipped_Log/1
  GNSS_Consume/3(last_epoch_out) -> GNSS_Last_Delivery/1
  GNSS_Last_Delivery/1 -> GNSS_Consume/3(last_epoch_in)
  GNSS_Poll_Clock/1 -> GNSS_Consume/2(time_s)
  GNSS_to_IMU/1 -> GNSS_Consume/1(packet)
  Receiver_Packet/1 -> GNSS_to_IMU/1

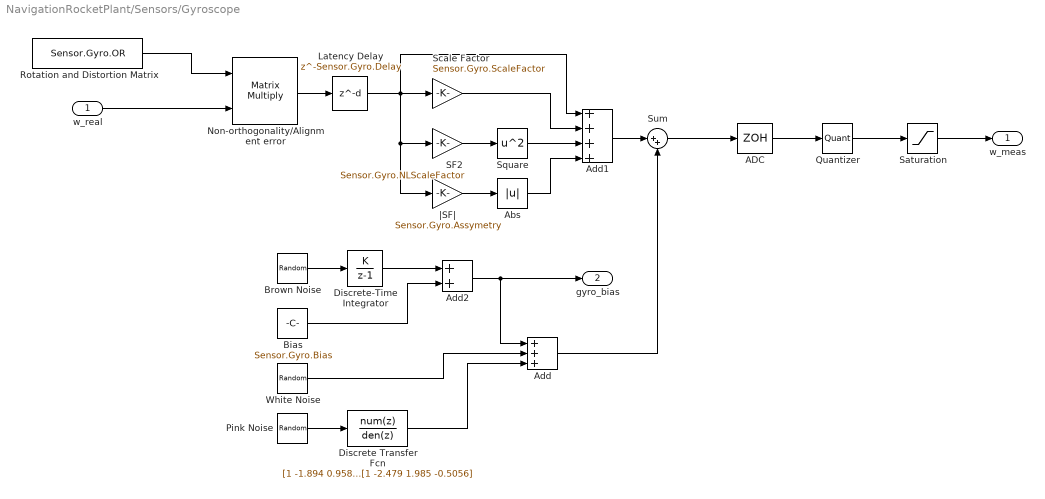
== system NavigationRocketPlant/Sensors/Gyroscope ==
  w_real : Inport
  ADC : ZeroOrderHold  SampleTime=Sensor.Gyro.Ts
  Abs : Abs  SaturateOnIntegerOverflow=off
  Add : Sum  Inputs=+++
  Add1 : Sum  Inputs=++++
  Add2 : Sum
  Bias : Constant  Value=Sensor.Gyro.Bias  VectorParams1D=off  SampleTime=Sensor.Gyro.Ts
  Brown Noise : RandomNumber  Mean=Sensor.Gyro.Noise.Brown.Mean  Variance=Sensor.Gyro.Noise.Brown.Variance  Seed=Sensor.Gyro.Noise.Brown.Seed  SampleTime=Sensor.Gyro.Ts  VectorParams1D=off
  Discrete Transfer Fcn : DiscreteTransferFcn  LoadFcn=dspblkCoreblockFVToolHelper(gcbh,'load');  Numerator=[1 -1.894 0.9586 -0.06213]  Denominator=[1 -2.479 1.985 -0.5056]
      settings: CopyFcn=dspblkCoreblockFVToolHelper(gcbh,'copy');  DeleteFcn=dspblkCoreblockFVToolHelper(gcbh,'close');  ModelCloseFcn=dspblkCoreblockFVToolHelper(gcbh,'close');  PreSaveFcn=dspblkCoreblockFVToolHelper(gcbh,'presave');  PostSaveFcn=dspblkCoreblockFVToolHelper(gcbh,'postsave');  CloseFcn=dspblkCoreblockFVToolHelper(gcbh,'close');
  Discrete-Time Integrator : DiscreteIntegrator  IntegratorMethod=Accumulation: Forward Euler  SampleTime=Sensor.Gyro.Ts  ICPrevOutput=DiscIntNeverNeededParam  ICPrevScaledInput=DiscIntNeverNeededParam
  Latency Delay : Delay  DelayLength=Sensor.Gyro.Delay  SampleTime=Sensor.Gyro.Ts
  Non-orthogonality/Alignment error : Product  Multiplication=Matrix(*)
  Pink Noise : RandomNumber  Mean=Sensor.Gyro.Noise.Pink.Mean  Variance=Sensor.Gyro.Noise.Pink.Variance  Seed=Sensor.Gyro.Noise.Pink.Seed  SampleTime=Sensor.Gyro.Ts  VectorParams1D=off
  Quantizer : Quantizer  QuantizationInterval=Sensor.Gyro.Quant
  Rotation and Distortion Matrix : Constant  Value=Sensor.Gyro.OR
  SF2 : Gain  Gain=Sensor.Gyro.NLScaleFactor
  "Saturation " : Saturate  UpperLimit=Sensor.Gyro.UpperLim  LowerLimit=Sensor.Gyro.LowerLim
  Scale Factor : Gain  Gain=Sensor.Gyro.ScaleFactor
  Square : Math  Operator=square
  Sum : Sum  Inputs=|++
  White Noise : RandomNumber  Mean=Sensor.Gyro.Noise.White.Mean  Variance=Sensor.Gyro.Noise.White.Variance  Seed=Sensor.Gyro.Noise.White.Seed  SampleTime=Sensor.Gyro.Ts  VectorParams1D=off
  |SF| : Gain  Gain=Sensor.Gyro.Assymetry
  w_meas : Outport
  gyro_bias : Outport  Port=2
  wires:
  w_real/1 -> Non-orthogonality/Alignment error/2
  Sum/1 -> ADC/1
  White Noise/1 -> Add/2
  Bias/1 -> Add2/2
  Add/1 -> Sum/2
  Brown Noise/1 -> Discrete-Time Integrator/1
  Discrete-Time Integrator/1 -> Add2/1
  ADC/1 -> Quantizer/1
  Latency Delay/1 -> Add1/1, SF2/1, |SF|/1, Scale Factor/1
  "Saturation "/1 -> w_meas/1
  Pink Noise/1 -> Discrete Transfer Fcn/1
  Discrete Transfer Fcn/1 -> Add/3
  SF2/1 -> Square/1
  |SF|/1 -> Abs/1
  Scale Factor/1 -> Add1/2
  Square/1 -> Add1/3
  Abs/1 -> Add1/4
  Add1/1 -> Sum/1
  Quantizer/1 -> "Saturation "/1
  Non-orthogonality/Alignment error/1 -> Latency Delay/1
  Rotation and Distortion Matrix/1 -> Non-orthogonality/Alignment error/1
  Add2/1 -> gyro_bias/1, Add/1

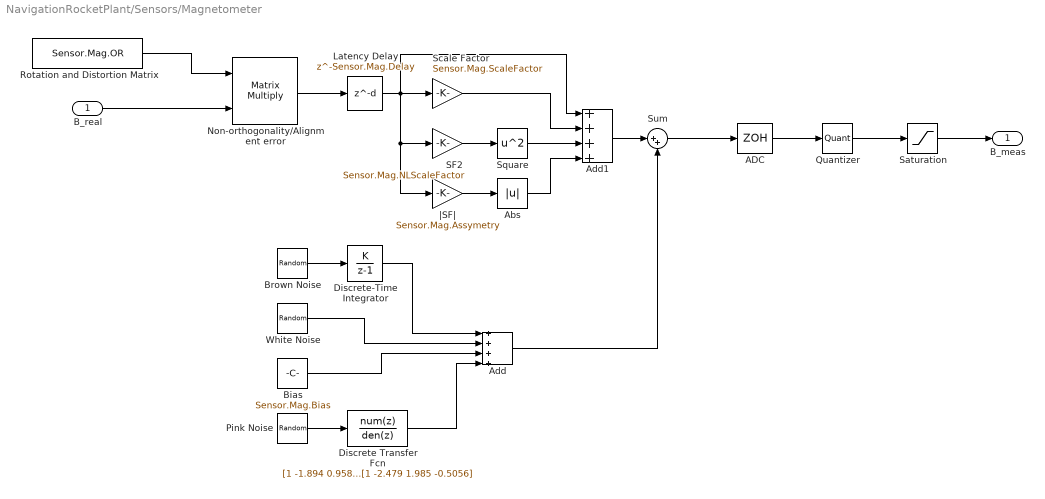
== system NavigationRocketPlant/Sensors/Magnetometer ==
  B_real : Inport
  ADC : ZeroOrderHold  SampleTime=Sensor.Mag.Ts
  Abs : Abs  SaturateOnIntegerOverflow=off
  Add : Sum  Inputs=++++
  Add1 : Sum  Inputs=++++
  Bias : Constant  Value=Sensor.Mag.Bias  VectorParams1D=off
  Brown Noise : RandomNumber  Mean=Sensor.Mag.Noise.Brown.Mean  Variance=Sensor.Mag.Noise.Brown.Variance  Seed=Sensor.Mag.Noise.Brown.Seed  SampleTime=Sensor.Mag.Ts  VectorParams1D=off
  Discrete Transfer Fcn : DiscreteTransferFcn  LoadFcn=dspblkCoreblockFVToolHelper(gcbh,'load');  Numerator=[1 -1.894 0.9586 -0.06213]  Denominator=[1 -2.479 1.985 -0.5056]
      settings: CopyFcn=dspblkCoreblockFVToolHelper(gcbh,'copy');  DeleteFcn=dspblkCoreblockFVToolHelper(gcbh,'close');  ModelCloseFcn=dspblkCoreblockFVToolHelper(gcbh,'close');  PreSaveFcn=dspblkCoreblockFVToolHelper(gcbh,'presave');  PostSaveFcn=dspblkCoreblockFVToolHelper(gcbh,'postsave');  CloseFcn=dspblkCoreblockFVToolHelper(gcbh,'close');
  Discrete-Time Integrator : DiscreteIntegrator  IntegratorMethod=Accumulation: Forward Euler  SampleTime=Sensor.Mag.Ts  ICPrevOutput=DiscIntNeverNeededParam  ICPrevScaledInput=DiscIntNeverNeededParam
  Latency Delay : Delay  DelayLength=Sensor.Mag.Delay  SampleTime=Sensor.Mag.Ts
  Non-orthogonality/Alignment error : Product  Multiplication=Matrix(*)
  Pink Noise : RandomNumber  Mean=Sensor.Mag.Noise.Pink.Mean  Variance=Sensor.Mag.Noise.Pink.Variance  Seed=Sensor.Mag.Noise.Pink.Seed  SampleTime=Sensor.Mag.Ts  VectorParams1D=off
  Quantizer : Quantizer  QuantizationInterval=Sensor.Mag.Quant
  Rotation and Distortion Matrix : Constant  Value=Sensor.Mag.OR
  SF2 : Gain  Gain=Sensor.Mag.NLScaleFactor
  "Saturation " : Saturate  UpperLimit=Sensor.Mag.UpperLim  LowerLimit=Sensor.Mag.LowerLim
  Scale Factor : Gain  Gain=Sensor.Mag.ScaleFactor
  Square : Math  Operator=square
  Sum : Sum  Inputs=|++
  White Noise : RandomNumber  Mean=Sensor.Mag.Noise.White.Mean  Variance=Sensor.Mag.Noise.White.Variance  Seed=Sensor.Mag.Noise.White.Seed  SampleTime=Sensor.Mag.Ts  VectorParams1D=off
  |SF| : Gain  Gain=Sensor.Mag.Assymetry
  B_meas : Outport
  wires:
  B_real/1 -> Non-orthogonality/Alignment error/2
  Sum/1 -> ADC/1
  White Noise/1 -> Add/2
  Bias/1 -> Add/3
  Add/1 -> Sum/2
  Brown Noise/1 -> Discrete-Time Integrator/1
  Discrete-Time Integrator/1 -> Add/1
  ADC/1 -> Quantizer/1
  Latency Delay/1 -> Add1/1, SF2/1, |SF|/1, Scale Factor/1
  "Saturation "/1 -> B_meas/1
  Pink Noise/1 -> Discrete Transfer Fcn/1
  Discrete Transfer Fcn/1 -> Add/4
  SF2/1 -> Square/1
  |SF|/1 -> Abs/1
  Scale Factor/1 -> Add1/2
  Square/1 -> Add1/3
  Abs/1 -> Add1/4
  Add1/1 -> Sum/1
  Quantizer/1 -> "Saturation "/1
  Non-orthogonality/Alignment error/1 -> Latency Delay/1
  Rotation and Distortion Matrix/1 -> Non-orthogonality/Alignment error/1

== system NavigationRocketPlant/Enviroment/System/Quaternion  ==
  wB : Inport
  A B|N : Subsystem
      settings: PortSchema="{\"entries\":[{\"content\":{\"sides\":[{\"content\":{},\"type\":\"ConnectorPlacement.EquallySpacedRectSide\",\"uuid\":\"4d96fdd9-76a2-4529-9825-527c636e83b2\"},{\"content\":{\"side\":\"RIGHT\"},\"type\":\"ConnectorPlacement.EquallySpacedRectSide\",\"uuid\":\"14690b11-ebf6-43a2-ba3f-2fb02211d3e0\"},{\"content\":{\"connectorIds\":[\"Out1\"],\"side\":\"TOP\"},\"type\":\"ConnectorPlacement.EquallySpacedRectSide\",\"uuid\":\"68905c31-32d1-4a49-b04d-ac4a34de50c9\"},{\"content\":{\"connectorIds\":[\"In1\"],\"side\":\"BOTTOM\"},\"type\":\"ConnectorPlacement.EquallySpacedRectSide\",\"uuid\":\"acf9cda8-e568-45e1-bc15-158d1d0dcbb8\"}]},\"type\":\"ConnectorPlacement.EquallySpacedConnector\",\"uuid\":\"abd9fe80-94ba-49ce-b6ad-d0e53bea3d6a\"}],\"packageUris\":[\"http://schema.mathworks.com/mf0/Connector/R2020b\"],\"version\":\"1.0\"}"
  Gain4 : Gain  Gain=1/2
  Integrator3 : Integrator  InitialCondition=q0
  Matrix Multiply7 : Product  Multiplication=Matrix(*)
  Normalization : dspmathops/Normalization  NormType=2-norm  Bias=1e-10  NormOver=Each column  Dimension=1  roundingMode=Floor  overflowMode=off  accumDataTypeStr=Inherit: Same as product output  accumLastDataTypeStr=Inherit: Same as product output  outputDataTypeStr=Inherit: Same as product output  outputMin=[]  outputMax=[]  outputLastDataTypeStr=Inherit: Same as product output
  Omega matrix : Subsystem
  q : Outport
  "A_B/N " : Outport  Port=2
  wires:
  Matrix Multiply7/1 -> Gain4/1
  Gain4/1 -> Integrator3/1  "q_dot"
  Integrator3/1 -> Normalization/1  "q"
  A B|N/1(A B|N) -> "A_B/N "/1  "A B|N"
  wB/1 -> Omega matrix/1(wB)
  Omega matrix/1(Om) -> Matrix Multiply7/1  "Om"
  Normalization/1 -> q/1, A B|N/1(q), Matrix Multiply7/2

== system NavigationRocketPlant/Enviroment/System/Quaternion /A B|N ==
  q : Inport
  Add : Sum  Inputs=+++
  Constant : Constant  Value=eye(3)
  Dot Product : DotProduct  OutDataTypeStr=Inherit: Inherit via internal rule
  Gain : Gain  Gain=2
  Gain1 : Gain  Gain=-2
  Matrix Multiply : Product
  Matrix Multiply1 : Product
  Matrix Multiply2 : Product  Multiplication=Matrix(*)
  Selector : Selector  InputPortWidth=4  IndexOptions=Index vector (dialog)  Indices=[4]  OutputSizes=1
  Selector1 : Selector  InputPortWidth=4  IndexOptions=Index vector (dialog)  Indices=[1:3]  OutputSizes=1
  Square : Math  Operator=square
  Subsystem : Subsystem
      settings: PortSchema="{\"entries\":[{\"content\":{\"sides\":[{\"content\":{},\"type\":\"ConnectorPlacement.EquallySpacedRectSide\",\"uuid\":\"4d96fdd9-76a2-4529-9825-527c636e83b2\"},{\"content\":{\"connectorIds\":[\"Out1\"],\"side\":\"RIGHT\"},\"type\":\"ConnectorPlacement.EquallySpacedRectSide\",\"uuid\":\"14690b11-ebf6-43a2-ba3f-2fb02211d3e0\"},{\"content\":{\"connectorIds\":[\"In1\"],\"side\":\"TOP\"},\"type\":\"ConnectorPlacement.EquallySpacedRectSide\",\"uuid\":\"68905c31-32d1-4a49-b04d-ac4a34de50c9\"}]},\"type\":\"ConnectorPlacement.EquallySpacedConnector\",\"uuid\":\"abd9fe80-94ba-49ce-b6ad-d0e53bea3d6a\"}],\"packageUris\":[\"http://schema.mathworks.com/mf0/Connector/R2020b\"],\"version\":\"1.0\"}"
  Sum : Sum  Inputs=+-|
  Transpose : Math  Operator=transpose
  A B|N : Outport
  wires:
  Add/1 -> A B|N/1  "A"
  Constant/1 -> Matrix Multiply/2
  Sum/1 -> Matrix Multiply/1
  q/1 -> Selector/1, Selector1/1  "q"
  Dot Product/1 -> Sum/2  "qqT"
  Transpose/1 -> Dot Product/1, Matrix Multiply2/2  "qT"
  Selector/1 -> Matrix Multiply1/1, Square/1  "q4"
  Square/1 -> Sum/1
  Matrix Multiply/1 -> Add/1
  Gain/1 -> Add/2
  Matrix Multiply1/1 -> Gain1/1
  Gain1/1 -> Add/3
  Subsystem/1(Out1) -> Matrix Multiply1/2  "[q^]"
  Selector1/1 -> Subsystem/1(q), Matrix Multiply2/1, Dot Product/2, Transpose/1
  Matrix Multiply2/1 -> Gain/1  "qqT"

== system NavigationRocketPlant/Enviroment/System/Quaternion /Omega matrix ==
  wB : Inport
  Constant1 : Constant  Value=0
  Demux : Demux  Outputs=3
  Gain : Gain  Gain=-1
  Gain1 : Gain  Gain=-1
  Gain2 : Gain  Gain=-1
  Reshape : Reshape  OutputDimensionality=Customize  OutputDimensions=[4,4]
  Vector Concatenate1 : Concatenate  NumInputs=16
  Om : Outport
  wires:
  wB/1 -> Demux/1  "w"
  Reshape/1 -> Om/1
  Constant1/1 -> Vector Concatenate1/1, Vector Concatenate1/6, Vector Concatenate1/11, Vector Concatenate1/16  "0"
  Demux/3 -> Vector Concatenate1/15, Vector Concatenate1/5, Gain/1  "wz"
  Gain/1 -> Vector Concatenate1/12, Vector Concatenate1/2  "-wz"
  Demux/2 -> Vector Concatenate1/14, Gain2/1, Vector Concatenate1/3  "wy"
  Demux/1 -> Gain1/1, Vector Concatenate1/10, Vector Concatenate1/13  "wx"
  Gain1/1 -> Vector Concatenate1/7, Vector Concatenate1/4  "-wx"
  Gain2/1 -> Vector Concatenate1/9, Vector Concatenate1/8  "-wy"
  Vector Concatenate1/1 -> Reshape/1

== system NavigationRocketPlant/Enviroment/System/Quaternion /A B|N/Subsystem ==
  q : Inport
  Constant : Constant  Value=0
  Demux : Demux  Outputs=3
  Gain : Gain  Gain=-1
  Gain1 : Gain  Gain=-1
  Gain2 : Gain  Gain=-1
  Reshape : Reshape  OutputDimensionality=Customize  OutputDimensions=[3,3]
  Vector Concatenate : Concatenate  NumInputs=9
  Out1 : Outport
  wires:
  Reshape/1 -> Out1/1  "[q^]"
  Vector Concatenate/1 -> Reshape/1
  Constant/1 -> Vector Concatenate/1, Vector Concatenate/9, Vector Concatenate/5
  Gain/1 -> Vector Concatenate/3
  Gain1/1 -> Vector Concatenate/4
  Gain2/1 -> Vector Concatenate/8
  q/1 -> Demux/1
  Demux/2 -> Vector Concatenate/7, Gain/1  "q2"
  Demux/3 -> Vector Concatenate/2, Gain1/1  "q3"
  Demux/1 -> Gain2/1, Vector Concatenate/6  "q1"

== matlab function NavigationRocketPlant/ISA Pressure to Altitude2 ==
  data: p input; h output
function h = ISA_pressure_to_altitude(p)

    % ISA pressure-to-altitude conversion for the troposphere.
    %
    % Input:
    %   p : static pressure [Pa]
    %
    % Output:
    %   h : altitude above sea level [m]
    %
    % Assumptions:
    %   - ISA troposphere model
    %   - sea-level pressure p0 = 101325 Pa
    %   - valid approximately for h < 11 km
    
    T0 = 288.15;       % sea-level standard temperature [K]
    L  = 0.0065;       % temperature lapse rate [K/m]
    R  = 287.05;       % specific gas constant for air [J/(kg K)]
    g0 = 9.80665;      % gravitational acceleration [m/s^2]
    p0 = 101325.0;     % sea-level standard pressure [Pa]
    
    exponent = (R * L) / g0;
    
    h = (T0 / L) * (1.0 - (p / p0)^exponent);

end

== matlab function NavigationRocketPlant/GNSS_LLA_to_NED ==
  data: llaDegM input; positionNED output; reference input; GNSSConfig parameter
function positionNED = GNSSLLAtoNED(llaDegM, reference, GNSSConfig)
% GPS output uses ellipsoid height. Restore the source altitude datum before
% conversion to local Down; never add the launch altitude a second time.
llaSourceDatum = llaDegM;
llaSourceDatum(3) = llaSourceDatum(3) - GNSSConfig.GeoidSeparation;
positionNED = gnssLlaToNed(llaSourceDatum, reference);
end
